simulink model "env_extQ32"  (R2022b)
settings: Solver=VariableStepAuto  StartTime=0.0  StopTime=30  RelTol=1e-3
values from neighbouring files (symbols this model uses):
  B = 8    [variables.m]    (also in variables16.m)
  cordic_delay = 20    [variables.m]    (also in variables16.m)
  e_val = 1/l2    [variables.m]    (also in variables16.m)
  exp_fract_len_homo = 26    [variables.m]    (also in variables16.m = 10)
  exp_word_len_homo = 32    [variables.m]    (also in variables16.m = 16)
  explarge_delay = 3    [variables.m]    (also in variables16.m)
  fft_len_hilb = 2048    [variables.m]    (also in variables16.m)
  fft_length = 4096    [variables.m]    (also in variables16.m)
  frac_bit_l2 = 30    [variables.m]    (also in variables16.m = 14)
  frac_bit_l3 = 29    [variables.m]    (also in variables16.m = 13)
  frac_bit_l4 = 28    [variables.m]    (also in variables16.m = 12)
  grp_delay_hilb = 11    [variables.m]    (also in variables16.m)
  grp_delay_homo = 13    [variables.m]    (also in variables16.m)
  grp_delay_psd = 19    [variables.m]    (also in variables16.m)
  grp_delay_swt = 12    [variables.m]    (also in variables16.m)
  l2 = log(2)    [variables.m]    (also in variables16.m)
  l2e = 1/log2(exp(1))    [variables.m]    (also in variables16.m)
  log2_table = log2((2^(B-1) : 2^(B)) / 2^(B - 1))    [variables.m]    (also in variables16.m)
  log_fract_len_homo = 31    [variables.m]    (also in variables16.m = 15)
  log_latency = 21    [variables.m]    (also in variables16.m)
  log_word_len = 48    [variables.m]    (also in variables16.m = 24)
  log_word_len_homo = 32    [variables.m]    (also in variables16.m = 16)
  NLZLUT = B-ceil(log2((1:2^B)))    [variables.m]    (also in variables16.m)
  scale = 1.0 / (fs * sum(window_val.*window_val))    [variables.m]    (also in variables16.m)
  win_dim = 64    [variables.m]    (also in variables16.m)
  window_dim = 100    [variables.m]    (also in variables16.m)
undefined symbols (not defined in the file or in its folder): c, fl_high_index, fl_low_index, HiD, hilbert_fifo_full, LoD, psd_fifo_full, sfvc784, swt_fifo_full, xck26, xlfda_numerator
libraries: hdlBasic x626, hdlDSPIP x12, hdlUtilities x2, dspsnks4 x1, dspvision x1, vmcUtilities x1
(part 6 of 7)

== system env_extQ32/env_extr/HOMOMORPHIC/log2/normalize_input/stage0 ==
  v_in : Inport
  mem_data_in : Inport  Port=2
  en : Inport  Port=3
  Delay1 : hdlBasic/Delay  rst=off  en=on  latency=1  reg_retiming=off  XmcBlockStatus=1  maskContainerNames=group1  block_type=delay  block_config=sysgen:Delay_config
  Mux : hdlBasic/Mux  inputs=9  en=on  latency=1  precision=Full  arith_type=Unsigned  n_bits=16  bin_pt=14  quantization=Truncate  overflow=Wrap  XmcBlockStatus=1  maskContainerNames=tabcontainer1  block_type=mux  block_config=sysgen:Mux_config
  Reinterpret : hdlBasic/Reinterpret  force_arith_type=on  arith_type=Unsigned  force_bin_pt=on  bin_pt=0  XmcBlockStatus=1  maskContainerNames=group1  block_type=reinterpret  block_config=sysgen:Reinterpret_config
  Shift1 : hdlBasic/Shift  shift_dir=Left  shift_bits=8  en=on  latency=1  precision=Full  arith_type="Signed  (2's comp)"  n_bits=16  bin_pt=14  quantization=Truncate  overflow=Wrap  XmcBlockStatus=1  maskContainerNames=group2  block_type=shift  block_config=sysgen:Shift_config
  Shift2 : hdlBasic/Shift  shift_dir=Left  shift_bits=1  en=on  latency=1  precision=Full  arith_type="Signed  (2's comp)"  n_bits=16  bin_pt=14  quantization=Truncate  overflow=Wrap  XmcBlockStatus=1  maskContainerNames=group2  block_type=shift  block_config=sysgen:Shift_config
  Shift3 : hdlBasic/Shift  shift_dir=Left  shift_bits=2  en=on  latency=1  precision=Full  arith_type="Signed  (2's comp)"  n_bits=16  bin_pt=14  quantization=Truncate  overflow=Wrap  XmcBlockStatus=1  maskContainerNames=group2  block_type=shift  block_config=sysgen:Shift_config
  Shift4 : hdlBasic/Shift  shift_dir=Left  shift_bits=3  en=on  latency=1  precision=Full  arith_type="Signed  (2's comp)"  n_bits=16  bin_pt=14  quantization=Truncate  overflow=Wrap  XmcBlockStatus=1  maskContainerNames=group2  block_type=shift  block_config=sysgen:Shift_config
  Shift5 : hdlBasic/Shift  shift_dir=Left  shift_bits=4  en=on  latency=1  precision=Full  arith_type="Signed  (2's comp)"  n_bits=16  bin_pt=14  quantization=Truncate  overflow=Wrap  XmcBlockStatus=1  maskContainerNames=group2  block_type=shift  block_config=sysgen:Shift_config
  Shift6 : hdlBasic/Shift  shift_dir=Left  shift_bits=5  en=on  latency=1  precision=Full  arith_type="Signed  (2's comp)"  n_bits=16  bin_pt=14  quantization=Truncate  overflow=Wrap  XmcBlockStatus=1  maskContainerNames=group2  block_type=shift  block_config=sysgen:Shift_config
  Shift7 : hdlBasic/Shift  shift_dir=Left  shift_bits=6  en=on  latency=1  precision=Full  arith_type="Signed  (2's comp)"  n_bits=16  bin_pt=14  quantization=Truncate  overflow=Wrap  XmcBlockStatus=1  maskContainerNames=group2  block_type=shift  block_config=sysgen:Shift_config
  Shift8 : hdlBasic/Shift  shift_dir=Left  shift_bits=7  en=on  latency=1  precision=Full  arith_type="Signed  (2's comp)"  n_bits=16  bin_pt=14  quantization=Truncate  overflow=Wrap  XmcBlockStatus=1  maskContainerNames=group2  block_type=shift  block_config=sysgen:Shift_config
  Shift9 : hdlBasic/Shift  shift_dir=Left  shift_bits=0  en=on  latency=1  precision=Full  arith_type="Signed  (2's comp)"  n_bits=16  bin_pt=14  quantization=Truncate  overflow=Wrap  XmcBlockStatus=1  maskContainerNames=group2  block_type=shift  block_config=sysgen:Shift_config
  Slice1 : hdlBasic/Slice  nbits=B  boolean_output=off  mode=Upper Bit Location + Width  bit1=0  base1=MSB of Input  bit0=8  base0=LSB of Input  XmcBlockStatus=1  maskContainerNames=group1  block_type=slice  block_config=sysgen:Slice_config
  v_out : Outport
  n_shift_out : Outport  Port=2
  mem_addr : Outport  Port=3
  wires:
  Shift7/1 -> Mux/8
  v_in/1 -> Reinterpret/1
  Shift4/1 -> Mux/5
  Shift6/1 -> Mux/7
  Shift2/1 -> Mux/3
  Shift8/1 -> Mux/9
  Shift3/1 -> Mux/4
  Shift5/1 -> Mux/6
  Delay1/1 -> n_shift_out/1
  Slice1/1 -> mem_addr/1
  Shift1/1 -> Mux/10
  Reinterpret/1 -> Shift1/1, Shift8/1, Shift7/1, Shift6/1, Shift5/1, Shift4/1, Shift3/1, Shift2/1, Shift9/1, Slice1/1
  Mux/1 -> v_out/1
  mem_data_in/1 -> Delay1/1, Mux/1
  Shift9/1 -> Mux/2
  en/1 -> Shift8/2, Shift7/2, Shift6/2, Shift5/2, Shift3/2, Shift2/2, Delay1/2, Mux/11, Shift9/2, Shift4/2, Shift1/2

== system env_extQ32/env_extr/HOMOMORPHIC/log2/normalize_input/stage1 ==
  v_in : Inport
  n_shift_in : Inport  Port=2
  mem_data_in : Inport  Port=3
  en : Inport  Port=4
  AddSub1 : hdlBasic/AddSub  mode=Addition  use_carryin=off  use_carryout=off  en=on  latency=1  precision=Full  arith_type=Unsigned  n_bits=16  bin_pt=14  quantization=Truncate  overflow=Wrap  use_behavioral_HDL=off  hw_selection=Fabric  pipelined=off  XmcBlockStatus=1  maskContainerNames=tabcontainer1  block_type=addsub  block_config=sysgen:Addsub_config
  Delay2 : hdlBasic/Delay  rst=off  en=on  latency=1  reg_retiming=off  XmcBlockStatus=1  maskContainerNames=group1  block_type=delay  block_config=sysgen:Delay_config
  Mux : hdlBasic/Mux  inputs=9  en=on  latency=1  precision=Full  arith_type=Unsigned  n_bits=16  bin_pt=14  quantization=Truncate  overflow=Wrap  XmcBlockStatus=1  maskContainerNames=tabcontainer1  block_type=mux  block_config=sysgen:Mux_config
  Shift1 : hdlBasic/Shift  shift_dir=Left  shift_bits=8  en=on  latency=1  precision=Full  arith_type="Signed  (2's comp)"  n_bits=16  bin_pt=14  quantization=Truncate  overflow=Wrap  XmcBlockStatus=1  maskContainerNames=group2  block_type=shift  block_config=sysgen:Shift_config
  Shift2 : hdlBasic/Shift  shift_dir=Left  shift_bits=1  en=on  latency=1  precision=Full  arith_type="Signed  (2's comp)"  n_bits=16  bin_pt=14  quantization=Truncate  overflow=Wrap  XmcBlockStatus=1  maskContainerNames=group2  block_type=shift  block_config=sysgen:Shift_config
  Shift3 : hdlBasic/Shift  shift_dir=Left  shift_bits=2  en=on  latency=1  precision=Full  arith_type="Signed  (2's comp)"  n_bits=16  bin_pt=14  quantization=Truncate  overflow=Wrap  XmcBlockStatus=1  maskContainerNames=group2  block_type=shift  block_config=sysgen:Shift_config
  Shift4 : hdlBasic/Shift  shift_dir=Left  shift_bits=3  en=on  latency=1  precision=Full  arith_type="Signed  (2's comp)"  n_bits=16  bin_pt=14  quantization=Truncate  overflow=Wrap  XmcBlockStatus=1  maskContainerNames=group2  block_type=shift  block_config=sysgen:Shift_config
  Shift5 : hdlBasic/Shift  shift_dir=Left  shift_bits=4  en=on  latency=1  precision=Full  arith_type="Signed  (2's comp)"  n_bits=16  bin_pt=14  quantization=Truncate  overflow=Wrap  XmcBlockStatus=1  maskContainerNames=group2  block_type=shift  block_config=sysgen:Shift_config
  Shift6 : hdlBasic/Shift  shift_dir=Left  shift_bits=5  en=on  latency=1  precision=Full  arith_type="Signed  (2's comp)"  n_bits=16  bin_pt=14  quantization=Truncate  overflow=Wrap  XmcBlockStatus=1  maskContainerNames=group2  block_type=shift  block_config=sysgen:Shift_config
  Shift7 : hdlBasic/Shift  shift_dir=Left  shift_bits=6  en=on  latency=1  precision=Full  arith_type="Signed  (2's comp)"  n_bits=16  bin_pt=14  quantization=Truncate  overflow=Wrap  XmcBlockStatus=1  maskContainerNames=group2  block_type=shift  block_config=sysgen:Shift_config
  Shift8 : hdlBasic/Shift  shift_dir=Left  shift_bits=7  en=on  latency=1  precision=Full  arith_type="Signed  (2's comp)"  n_bits=16  bin_pt=14  quantization=Truncate  overflow=Wrap  XmcBlockStatus=1  maskContainerNames=group2  block_type=shift  block_config=sysgen:Shift_config
  Shift9 : hdlBasic/Shift  shift_dir=Left  shift_bits=0  en=on  latency=1  precision=Full  arith_type="Signed  (2's comp)"  n_bits=16  bin_pt=14  quantization=Truncate  overflow=Wrap  XmcBlockStatus=1  maskContainerNames=group2  block_type=shift  block_config=sysgen:Shift_config
  Slice1 : hdlBasic/Slice  nbits=B  boolean_output=off  mode=Upper Bit Location + Width  bit1=0  base1=MSB of Input  bit0=8  base0=LSB of Input  XmcBlockStatus=1  maskContainerNames=group1  block_type=slice  block_config=sysgen:Slice_config
  v_out : Outport
  n_shift_out : Outport  Port=2
  mem_addr : Outport  Port=3
  wires:
  Shift7/1 -> Mux/8
  Shift4/1 -> Mux/5
  Shift6/1 -> Mux/7
  Shift2/1 -> Mux/3
  Shift8/1 -> Mux/9
  Shift3/1 -> Mux/4
  Shift5/1 -> Mux/6
  Slice1/1 -> mem_addr/1
  Shift1/1 -> Mux/10
  v_in/1 -> Shift1/1, Shift8/1, Shift7/1, Shift6/1, Shift5/1, Shift4/1, Shift3/1, Shift2/1, Shift9/1, Slice1/1
  Mux/1 -> v_out/1
  AddSub1/1 -> n_shift_out/1
  n_shift_in/1 -> Delay2/1
  mem_data_in/1 -> AddSub1/2, Mux/1
  Delay2/1 -> AddSub1/1
  Shift9/1 -> Mux/2
  en/1 -> Shift8/2, Shift7/2, Shift6/2, Shift5/2, Shift4/2, Shift3/2, Shift2/2, Mux/11, AddSub1/3, Delay2/2, Shift9/2, Shift1/2

== system env_extQ32/env_extr/HOMOMORPHIC/log2/normalize_input/stage2 ==
  v_in : Inport
  n_shift_in : Inport  Port=2
  mem_data_in : Inport  Port=3
  en : Inport  Port=4
  AddSub1 : hdlBasic/AddSub  mode=Addition  use_carryin=off  use_carryout=off  en=on  latency=1  precision=Full  arith_type=Unsigned  n_bits=16  bin_pt=14  quantization=Truncate  overflow=Wrap  use_behavioral_HDL=off  hw_selection=Fabric  pipelined=off  XmcBlockStatus=1  maskContainerNames=tabcontainer1  block_type=addsub  block_config=sysgen:Addsub_config
  Delay2 : hdlBasic/Delay  rst=off  en=on  latency=1  reg_retiming=off  XmcBlockStatus=1  maskContainerNames=group1  block_type=delay  block_config=sysgen:Delay_config
  Mux : hdlBasic/Mux  inputs=9  en=on  latency=1  precision=Full  arith_type=Unsigned  n_bits=16  bin_pt=14  quantization=Truncate  overflow=Wrap  XmcBlockStatus=1  maskContainerNames=tabcontainer1  block_type=mux  block_config=sysgen:Mux_config
  Shift1 : hdlBasic/Shift  shift_dir=Left  shift_bits=8  en=on  latency=1  precision=Full  arith_type="Signed  (2's comp)"  n_bits=16  bin_pt=14  quantization=Truncate  overflow=Wrap  XmcBlockStatus=1  maskContainerNames=group2  block_type=shift  block_config=sysgen:Shift_config
  Shift2 : hdlBasic/Shift  shift_dir=Left  shift_bits=1  en=on  latency=1  precision=Full  arith_type="Signed  (2's comp)"  n_bits=16  bin_pt=14  quantization=Truncate  overflow=Wrap  XmcBlockStatus=1  maskContainerNames=group2  block_type=shift  block_config=sysgen:Shift_config
  Shift3 : hdlBasic/Shift  shift_dir=Left  shift_bits=2  en=on  latency=1  precision=Full  arith_type="Signed  (2's comp)"  n_bits=16  bin_pt=14  quantization=Truncate  overflow=Wrap  XmcBlockStatus=1  maskContainerNames=group2  block_type=shift  block_config=sysgen:Shift_config
  Shift4 : hdlBasic/Shift  shift_dir=Left  shift_bits=3  en=on  latency=1  precision=Full  arith_type="Signed  (2's comp)"  n_bits=16  bin_pt=14  quantization=Truncate  overflow=Wrap  XmcBlockStatus=1  maskContainerNames=group2  block_type=shift  block_config=sysgen:Shift_config
  Shift5 : hdlBasic/Shift  shift_dir=Left  shift_bits=4  en=on  latency=1  precision=Full  arith_type="Signed  (2's comp)"  n_bits=16  bin_pt=14  quantization=Truncate  overflow=Wrap  XmcBlockStatus=1  maskContainerNames=group2  block_type=shift  block_config=sysgen:Shift_config
  Shift6 : hdlBasic/Shift  shift_dir=Left  shift_bits=5  en=on  latency=1  precision=Full  arith_type="Signed  (2's comp)"  n_bits=16  bin_pt=14  quantization=Truncate  overflow=Wrap  XmcBlockStatus=1  maskContainerNames=group2  block_type=shift  block_config=sysgen:Shift_config
  Shift7 : hdlBasic/Shift  shift_dir=Left  shift_bits=6  en=on  latency=1  precision=Full  arith_type="Signed  (2's comp)"  n_bits=16  bin_pt=14  quantization=Truncate  overflow=Wrap  XmcBlockStatus=1  maskContainerNames=group2  block_type=shift  block_config=sysgen:Shift_config
  Shift8 : hdlBasic/Shift  shift_dir=Left  shift_bits=7  en=on  latency=1  precision=Full  arith_type="Signed  (2's comp)"  n_bits=16  bin_pt=14  quantization=Truncate  overflow=Wrap  XmcBlockStatus=1  maskContainerNames=group2  block_type=shift  block_config=sysgen:Shift_config
  Shift9 : hdlBasic/Shift  shift_dir=Left  shift_bits=0  en=on  latency=1  precision=Full  arith_type="Signed  (2's comp)"  n_bits=16  bin_pt=14  quantization=Truncate  overflow=Wrap  XmcBlockStatus=1  maskContainerNames=group2  block_type=shift  block_config=sysgen:Shift_config
  Slice1 : hdlBasic/Slice  nbits=B  boolean_output=off  mode=Upper Bit Location + Width  bit1=0  base1=MSB of Input  bit0=8  base0=LSB of Input  XmcBlockStatus=1  maskContainerNames=group1  block_type=slice  block_config=sysgen:Slice_config
  v_out : Outport
  n_shift_out : Outport  Port=2
  mem_addr : Outport  Port=3
  wires:
  Shift7/1 -> Mux/8
  Shift4/1 -> Mux/5
  Shift6/1 -> Mux/7
  Shift2/1 -> Mux/3
  Shift8/1 -> Mux/9
  Shift3/1 -> Mux/4
  Shift5/1 -> Mux/6
  Slice1/1 -> mem_addr/1
  Shift1/1 -> Mux/10
  v_in/1 -> Shift1/1, Shift8/1, Shift7/1, Shift6/1, Shift5/1, Shift4/1, Shift3/1, Shift2/1, Shift9/1, Slice1/1
  Mux/1 -> v_out/1
  AddSub1/1 -> n_shift_out/1
  n_shift_in/1 -> Delay2/1
  mem_data_in/1 -> AddSub1/2, Mux/1
  Delay2/1 -> AddSub1/1
  Shift9/1 -> Mux/2
  en/1 -> Shift8/2, Shift7/2, Shift6/2, Shift5/2, Shift4/2, Shift3/2, Shift2/2, Delay2/2, Mux/11, AddSub1/3, Shift9/2, Shift1/2

== system env_extQ32/env_extr/HOMOMORPHIC/log2/normalize_input/stage3 ==
  v_in : Inport
  n_shift_in : Inport  Port=2
  mem_data_in : Inport  Port=3
  en : Inport  Port=4
  AddSub1 : hdlBasic/AddSub  mode=Subtraction  use_carryin=off  use_carryout=off  en=on  latency=1  precision=Full  arith_type=Unsigned  n_bits=16  bin_pt=14  quantization=Truncate  overflow=Wrap  use_behavioral_HDL=off  hw_selection=Fabric  pipelined=off  XmcBlockStatus=1  maskContainerNames=tabcontainer1  block_type=addsub  block_config=sysgen:Addsub_config
  AddSub2 : hdlBasic/AddSub  mode=Subtraction  use_carryin=off  use_carryout=off  en=on  latency=1  precision=Full  arith_type=Unsigned  n_bits=16  bin_pt=14  quantization=Truncate  overflow=Wrap  use_behavioral_HDL=off  hw_selection=Fabric  pipelined=off  XmcBlockStatus=1  maskContainerNames=tabcontainer1  block_type=addsub  block_config=sysgen:Addsub_config
  Constant1 : hdlBasic/Constant  const=log_word_len_homo-log_fract_len_homo-1  gui_display_data_type=Fixed-point  arith_type=Unsigned  n_bits=ceil(log2(log_word_len_homo-log_fract_len_homo+1))  bin_pt=0  preci_type=Single  exp_width=8  frac_width=24  explicit_period=off  period=1  XmcBlockStatus=1  maskContainerNames=tabcontainer1  block_type=constant  block_config=sysgen:Constant_config
  Mux : hdlBasic/Mux  inputs=9  en=on  latency=1  precision=Full  arith_type=Unsigned  n_bits=16  bin_pt=14  quantization=Truncate  overflow=Wrap  XmcBlockStatus=1  maskContainerNames=tabcontainer1  block_type=mux  block_config=sysgen:Mux_config
  Reinterpret : hdlBasic/Reinterpret  force_arith_type=off  arith_type=Unsigned  force_bin_pt=on  bin_pt=log_word_len_homo-1  XmcBlockStatus=1  maskContainerNames=group1  block_type=reinterpret  block_config=sysgen:Reinterpret_config
  Shift1 : hdlBasic/Shift  shift_dir=Left  shift_bits=8  en=on  latency=1  precision=Full  arith_type="Signed  (2's comp)"  n_bits=16  bin_pt=14  quantization=Truncate  overflow=Wrap  XmcBlockStatus=1  maskContainerNames=group2  block_type=shift  block_config=sysgen:Shift_config
  Shift2 : hdlBasic/Shift  shift_dir=Left  shift_bits=1  en=on  latency=1  precision=Full  arith_type="Signed  (2's comp)"  n_bits=16  bin_pt=14  quantization=Truncate  overflow=Wrap  XmcBlockStatus=1  maskContainerNames=group2  block_type=shift  block_config=sysgen:Shift_config
  Shift3 : hdlBasic/Shift  shift_dir=Left  shift_bits=2  en=on  latency=1  precision=Full  arith_type="Signed  (2's comp)"  n_bits=16  bin_pt=14  quantization=Truncate  overflow=Wrap  XmcBlockStatus=1  maskContainerNames=group2  block_type=shift  block_config=sysgen:Shift_config
  Shift4 : hdlBasic/Shift  shift_dir=Left  shift_bits=3  en=on  latency=1  precision=Full  arith_type="Signed  (2's comp)"  n_bits=16  bin_pt=14  quantization=Truncate  overflow=Wrap  XmcBlockStatus=1  maskContainerNames=group2  block_type=shift  block_config=sysgen:Shift_config
  Shift5 : hdlBasic/Shift  shift_dir=Left  shift_bits=4  en=on  latency=1  precision=Full  arith_type="Signed  (2's comp)"  n_bits=16  bin_pt=14  quantization=Truncate  overflow=Wrap  XmcBlockStatus=1  maskContainerNames=group2  block_type=shift  block_config=sysgen:Shift_config
  Shift6 : hdlBasic/Shift  shift_dir=Left  shift_bits=5  en=on  latency=1  precision=Full  arith_type="Signed  (2's comp)"  n_bits=16  bin_pt=14  quantization=Truncate  overflow=Wrap  XmcBlockStatus=1  maskContainerNames=group2  block_type=shift  block_config=sysgen:Shift_config
  Shift7 : hdlBasic/Shift  shift_dir=Left  shift_bits=6  en=on  latency=1  precision=Full  arith_type="Signed  (2's comp)"  n_bits=16  bin_pt=14  quantization=Truncate  overflow=Wrap  XmcBlockStatus=1  maskContainerNames=group2  block_type=shift  block_config=sysgen:Shift_config
  Shift8 : hdlBasic/Shift  shift_dir=Left  shift_bits=7  en=on  latency=1  precision=Full  arith_type="Signed  (2's comp)"  n_bits=16  bin_pt=14  quantization=Truncate  overflow=Wrap  XmcBlockStatus=1  maskContainerNames=group2  block_type=shift  block_config=sysgen:Shift_config
  Shift9 : hdlBasic/Shift  shift_dir=Left  shift_bits=0  en=on  latency=1  precision=Full  arith_type="Signed  (2's comp)"  n_bits=16  bin_pt=14  quantization=Truncate  overflow=Wrap  XmcBlockStatus=1  maskContainerNames=group2  block_type=shift  block_config=sysgen:Shift_config
  Slice1 : hdlBasic/Slice  nbits=B  boolean_output=off  mode=Upper Bit Location + Width  bit1=0  base1=MSB of Input  bit0=8  base0=LSB of Input  XmcBlockStatus=1  maskContainerNames=group1  block_type=slice  block_config=sysgen:Slice_config
  v_out : Outport
  n_shift_out : Outport  Port=2
  mem_addr : Outport  Port=3
  wires:
  Shift7/1 -> Mux/8
  Shift4/1 -> Mux/5
  Shift6/1 -> Mux/7
  Shift2/1 -> Mux/3
  Shift8/1 -> Mux/9
  Shift3/1 -> Mux/4
  Shift5/1 -> Mux/6
  Mux/1 -> Reinterpret/1
  n_shift_in/1 -> AddSub2/2
  AddSub2/1 -> AddSub1/1
  Constant1/1 -> AddSub2/1
  mem_data_in/1 -> AddSub1/2, Mux/1
  v_in/1 -> Slice1/1, Shift1/1, Shift8/1, Shift7/1, Shift6/1, Shift5/1, Shift4/1, Shift3/1, Shift2/1, Shift9/1
  Slice1/1 -> mem_addr/1
  Reinterpret/1 -> v_out/1
  Shift1/1 -> Mux/10
  AddSub1/1 -> n_shift_out/1
  Shift9/1 -> Mux/2
  en/1 -> Shift8/2, Shift7/2, Shift6/2, Shift5/2, Shift4/2, Shift3/2, Shift2/2, AddSub2/3, Mux/11, AddSub1/3, Shift9/2, Shift1/2

== system env_extQ32/env_extr/SWT/shannonE/log2/normalize_input ==
  data_in : Inport
  en : Inport  Port=2
  Constant1 : hdlBasic/Constant  const=0  gui_display_data_type=Boolean  arith_type=Boolean  n_bits=16  bin_pt=14  preci_type=Single  exp_width=8  frac_width=24  explicit_period=off  period=1  XmcBlockStatus=1  maskContainerNames=tabcontainer1  block_type=constant  block_config=sysgen:Constant_config
  Constant2 : hdlBasic/Constant  const=0  gui_display_data_type=Boolean  arith_type=Boolean  n_bits=16  bin_pt=14  preci_type=Single  exp_width=8  frac_width=24  explicit_period=off  period=1  XmcBlockStatus=1  maskContainerNames=tabcontainer1  block_type=constant  block_config=sysgen:Constant_config
  Constant3 : hdlBasic/Constant  const=0  gui_display_data_type=Fixed-point  arith_type=Unsigned  n_bits=ceil(log2(B)+1)  bin_pt=0  preci_type=Single  exp_width=8  frac_width=24  explicit_period=off  period=1  XmcBlockStatus=1  maskContainerNames=tabcontainer1  block_type=constant  block_config=sysgen:Constant_config
  Constant4 : hdlBasic/Constant  const=0  gui_display_data_type=Fixed-point  arith_type=Unsigned  n_bits=ceil(log2(B)+1)  bin_pt=0  preci_type=Single  exp_width=8  frac_width=24  explicit_period=off  period=1  XmcBlockStatus=1  maskContainerNames=tabcontainer1  block_type=constant  block_config=sysgen:Constant_config
  Constant7 : hdlBasic/Constant  const=0  gui_display_data_type=Boolean  arith_type=Boolean  n_bits=16  bin_pt=14  preci_type=Single  exp_width=8  frac_width=24  explicit_period=off  period=1  XmcBlockStatus=1  maskContainerNames=tabcontainer1  block_type=constant  block_config=sysgen:Constant_config
  Constant8 : hdlBasic/Constant  const=0  gui_display_data_type=Fixed-point  arith_type=Unsigned  n_bits=ceil(log2(B)+1)  bin_pt=0  preci_type=Single  exp_width=8  frac_width=24  explicit_period=off  period=1  XmcBlockStatus=1  maskContainerNames=tabcontainer1  block_type=constant  block_config=sysgen:Constant_config
  Dual Port RAM : hdlBasic/Dual Port RAM  depth=length(NLZLUT)  initVector=NLZLUT  distributed_mem=Block RAM  init_a=0  init_b=0  rst_a=off  rst_b=off  en_a=on  en_b=on  latency=1  write_mode_A=Read After Write  write_mode_B=Read After Write  explicit_period=[]  period=[]  simulation_type=fast_sim  XmcBlockStatus=1  maskContainerNames=tabcontainer1  block_type=dpram  block_config=sysgen:Dpram_config  optimize=Area
      settings: infoedit=[]
  Dual Port RAM1 : hdlBasic/Dual Port RAM  depth=length(NLZLUT)  initVector=NLZLUT  distributed_mem=Block RAM  init_a=0  init_b=0  rst_a=off  rst_b=off  en_a=on  en_b=on  latency=1  write_mode_A=Read After Write  write_mode_B=Read After Write  explicit_period=[]  period=[]  simulation_type=fast_sim  XmcBlockStatus=1  maskContainerNames=tabcontainer1  block_type=dpram  block_config=sysgen:Dpram_config  optimize=Area
      settings: infoedit=[]
  Dual Port RAM3 : hdlBasic/Dual Port RAM  depth=length(NLZLUT)  initVector=NLZLUT  distributed_mem=Block RAM  init_a=0  init_b=0  rst_a=off  rst_b=off  en_a=on  en_b=on  latency=1  write_mode_A=Read After Write  write_mode_B=Read After Write  explicit_period=[]  period=[]  simulation_type=fast_sim  XmcBlockStatus=1  maskContainerNames=tabcontainer1  block_type=dpram  block_config=sysgen:Dpram_config  optimize=Area
      settings: infoedit=[]
  stage0 : Subsystem
      settings: PortSchema="{\"entries\":[{\"content\":{\"sides\":[{\"content\":{\"connectorIds\":[\"In1\"]},\"type\":\"ConnectorPlacement.EquallySpacedRectSide\",\"uuid\":\"2efcf317-0d6c-449c-9b5f-ecffd8c2580d\"},{\"content\":{\"connectorIds\":[\"Out1\",\"Out2\"],\"side\":\"RIGHT\"},\"type\":\"ConnectorPlacement.EquallySpacedRectSide\",\"uuid\":\"64d64660-0707-42f2-9c9c-1ef5504f52ac\"},{\"content\":{\"connectorIds\":[\"In2\",\"In3\",\"Out3\"],\"side\":\"TOP\"},\"type\":\"ConnectorPlacement.EquallySpacedRectSide\",\"uuid\":\"46f06ac4-fdd0-4e37-81b8-c7ff4ab208c3\"}]},\"type\":\"ConnectorPlacement.EquallySpacedConnector\",\"uuid\":\"22d944fc-118c-4e93-8f45-ec21c3a091f8\"}],\"packageUris\":[\"http://schema.mathworks.com/mf0/Connector/R2020b\"],\"version\":\"1.0\"}"
  stage1 : Subsystem
      settings: PortSchema="{\"entries\":[{\"content\":{\"sides\":[{\"content\":{\"connectorIds\":[\"In1\",\"In2\"]},\"type\":\"ConnectorPlacement.EquallySpacedRectSide\",\"uuid\":\"9d039a16-3a48-49d5-80b7-ade04a8e7f96\"},{\"content\":{\"connectorIds\":[\"Out1\",\"Out2\"],\"side\":\"RIGHT\"},\"type\":\"ConnectorPlacement.EquallySpacedRectSide\",\"uuid\":\"bb4be220-296c-4d2d-b90e-a958a467eb47\"},{\"content\":{\"connectorIds\":[\"In3\",\"In4\",\"Out3\"],\"side\":\"TOP\"},\"type\":\"ConnectorPlacement.EquallySpacedRectSide\",\"uuid\":\"bb4a24ca-25c4-4b34-8f6b-74df8c85655a\"}]},\"type\":\"ConnectorPlacement.EquallySpacedConnector\",\"uuid\":\"a2ca7259-7cd6-4f5b-b082-7ba40fce56a8\"}],\"packageUris\":[\"http://schema.mathworks.com/mf0/Connector/R2020b\"],\"version\":\"1.0\"}"
  stage2 : Subsystem
      settings: PortSchema="{\"entries\":[{\"content\":{\"sides\":[{\"content\":{\"connectorIds\":[\"In1\",\"In2\"]},\"type\":\"ConnectorPlacement.EquallySpacedRectSide\",\"uuid\":\"9d039a16-3a48-49d5-80b7-ade04a8e7f96\"},{\"content\":{\"connectorIds\":[\"Out1\",\"Out2\"],\"side\":\"RIGHT\"},\"type\":\"ConnectorPlacement.EquallySpacedRectSide\",\"uuid\":\"bb4be220-296c-4d2d-b90e-a958a467eb47\"},{\"content\":{\"connectorIds\":[\"In3\",\"In4\",\"Out3\"],\"side\":\"TOP\"},\"type\":\"ConnectorPlacement.EquallySpacedRectSide\",\"uuid\":\"bb4a24ca-25c4-4b34-8f6b-74df8c85655a\"}]},\"type\":\"ConnectorPlacement.EquallySpacedConnector\",\"uuid\":\"a2ca7259-7cd6-4f5b-b082-7ba40fce56a8\"}],\"packageUris\":[\"http://schema.mathworks.com/mf0/Connector/R2020b\"],\"version\":\"1.0\"}"
  stage3 : Subsystem
      settings: PortSchema="{\"entries\":[{\"content\":{\"sides\":[{\"content\":{\"connectorIds\":[\"In1\",\"In2\"]},\"type\":\"ConnectorPlacement.EquallySpacedRectSide\",\"uuid\":\"9d039a16-3a48-49d5-80b7-ade04a8e7f96\"},{\"content\":{\"connectorIds\":[\"Out1\",\"Out2\"],\"side\":\"RIGHT\"},\"type\":\"ConnectorPlacement.EquallySpacedRectSide\",\"uuid\":\"bb4be220-296c-4d2d-b90e-a958a467eb47\"},{\"content\":{\"connectorIds\":[\"In3\",\"In4\",\"Out3\"],\"side\":\"TOP\"},\"type\":\"ConnectorPlacement.EquallySpacedRectSide\",\"uuid\":\"bb4a24ca-25c4-4b34-8f6b-74df8c85655a\"}]},\"type\":\"ConnectorPlacement.EquallySpacedConnector\",\"uuid\":\"a2ca7259-7cd6-4f5b-b082-7ba40fce56a8\"}],\"packageUris\":[\"http://schema.mathworks.com/mf0/Connector/R2020b\"],\"version\":\"1.0\"}"
  stage7 : Subsystem
      settings: PortSchema="{\"entries\":[{\"content\":{\"sides\":[{\"content\":{\"connectorIds\":[\"In1\",\"In2\"]},\"type\":\"ConnectorPlacement.EquallySpacedRectSide\",\"uuid\":\"9d039a16-3a48-49d5-80b7-ade04a8e7f96\"},{\"content\":{\"connectorIds\":[\"Out1\",\"Out2\"],\"side\":\"RIGHT\"},\"type\":\"ConnectorPlacement.EquallySpacedRectSide\",\"uuid\":\"bb4be220-296c-4d2d-b90e-a958a467eb47\"},{\"content\":{\"connectorIds\":[\"In3\",\"In4\",\"Out3\"],\"side\":\"TOP\"},\"type\":\"ConnectorPlacement.EquallySpacedRectSide\",\"uuid\":\"bb4a24ca-25c4-4b34-8f6b-74df8c85655a\"}]},\"type\":\"ConnectorPlacement.EquallySpacedConnector\",\"uuid\":\"a2ca7259-7cd6-4f5b-b082-7ba40fce56a8\"}],\"packageUris\":[\"http://schema.mathworks.com/mf0/Connector/R2020b\"],\"version\":\"1.0\"}"
  stage8 : Subsystem
      settings: PortSchema="{\"entries\":[{\"content\":{\"sides\":[{\"content\":{\"connectorIds\":[\"In1\",\"In2\"]},\"type\":\"ConnectorPlacement.EquallySpacedRectSide\",\"uuid\":\"f634d078-23dc-4ab7-95a0-12deec3a8dc3\"},{\"content\":{\"connectorIds\":[\"Out1\",\"Out2\"],\"side\":\"RIGHT\"},\"type\":\"ConnectorPlacement.EquallySpacedRectSide\",\"uuid\":\"3b518452-2987-4406-a2e9-8ddbf9d6e9f5\"},{\"content\":{\"connectorIds\":[\"In3\",\"In4\",\"Out3\"],\"side\":\"TOP\"},\"type\":\"ConnectorPlacement.EquallySpacedRectSide\",\"uuid\":\"9ad2e8b0-6de8-48f9-a4db-ba88e5ff6307\"}]},\"type\":\"ConnectorPlacement.EquallySpacedConnector\",\"uuid\":\"bfdc1522-4211-4337-893d-197f1173dc35\"}],\"packageUris\":[\"http://schema.mathworks.com/mf0/Connector/R2020b\"],\"version\":\"1.0\"}"
  data_out_x : Outport
  data_out_n : Outport  Port=2
  wires:
  stage8/1(v_out) -> data_out_x/1
  stage8/2(n_shift_out) -> data_out_n/1
  stage7/1(v_out) -> stage8/1(v_in)
  stage7/2(n_shift_out) -> stage8/2(n_shift_in)
  data_in/1 -> stage0/1(v_in)
  stage0/1(v_out) -> stage1/1(v_in)
  stage0/2(n_shift_out) -> stage1/2(n_shift_in)
  Constant2/1 -> Dual Port RAM/3, Dual Port RAM/6
  Constant3/1 -> Dual Port RAM/2, Dual Port RAM/5
  Dual Port RAM/1 -> stage0/2(mem_data_in)  "log2lut"
  stage0/3(mem_addr) -> Dual Port RAM/1
  Dual Port RAM/2 -> stage1/3(mem_data_in)  "log2luti1"
  stage1/3(mem_addr) -> Dual Port RAM/4
  Constant7/1 -> Dual Port RAM3/3, Dual Port RAM3/6
  Constant8/1 -> Dual Port RAM3/5, Dual Port RAM3/2
  Dual Port RAM3/2 -> stage7/3(mem_data_in)  "log2luti1"
  stage7/3(mem_addr) -> Dual Port RAM3/4
  Dual Port RAM3/1 -> stage8/3(mem_data_in)  "log2lut"
  stage8/3(mem_addr) -> Dual Port RAM3/1
  stage2/1(v_out) -> stage3/1(v_in)
  stage2/2(n_shift_out) -> stage3/2(n_shift_in)
  stage1/1(v_out) -> stage2/1(v_in)
  stage1/2(n_shift_out) -> stage2/2(n_shift_in)
  stage3/2(n_shift_out) -> stage7/2(n_shift_in)
  stage3/1(v_out) -> stage7/1(v_in)
  en/1 -> Dual Port RAM1/8, Dual Port RAM1/7, stage3/4(en), stage7/4(en), Dual Port RAM3/8, Dual Port RAM3/7, stage8/4(en), stage2/4(en), stage1/4(en), Dual Port RAM/8, Dual Port RAM/7, stage0/3(en)
  Constant4/1 -> Dual Port RAM1/2, Dual Port RAM1/5
  Constant1/1 -> Dual Port RAM1/3, Dual Port RAM1/6
  stage2/3(mem_addr) -> Dual Port RAM1/1
  Dual Port RAM1/1 -> stage2/3(mem_data_in)  "log2lut"
  Dual Port RAM1/2 -> stage3/3(mem_data_in)  "log2luti1"
  stage3/3(mem_addr) -> Dual Port RAM1/4

== system env_extQ32/env_extr/SWT/shannonE/log2/normalize_input/stage0 ==
  v_in : Inport
  mem_data_in : Inport  Port=2
  en : Inport  Port=3
  Delay1 : hdlBasic/Delay  rst=off  en=on  latency=1  reg_retiming=off  XmcBlockStatus=1  maskContainerNames=group1  block_type=delay  block_config=sysgen:Delay_config
  Mux : hdlBasic/Mux  inputs=9  en=on  latency=1  precision=Full  arith_type=Unsigned  n_bits=16  bin_pt=14  quantization=Truncate  overflow=Wrap  XmcBlockStatus=1  maskContainerNames=tabcontainer1  block_type=mux  block_config=sysgen:Mux_config
  ROM : hdlBasic/ROM  Commented=on  depth=length(NLZLUT)  initVector=NLZLUT  distributed_mem=Block RAM  rst=off  init_reg=0  en=off  latency=1  gui_display_data_type=Fixed-point  arith_type=Unsigned  n_bits=ceil(log2(B)+1)  bin_pt=0  preci_type=Single  exp_width=8  frac_width=24  optimize=Area  use_rpm=on  simulation_type=fast_sim  XmcBlockStatus=1  maskContainerNames=tabcontainer1  block_type=sprom  block_config=sysgen:SPROM_config
  Reinterpret : hdlBasic/Reinterpret  force_arith_type=on  arith_type=Unsigned  force_bin_pt=on  bin_pt=0  XmcBlockStatus=1  maskContainerNames=group1  block_type=reinterpret  block_config=sysgen:Reinterpret_config
  Shift1 : hdlBasic/Shift  shift_dir=Left  shift_bits=8  en=on  latency=1  precision=Full  arith_type="Signed  (2's comp)"  n_bits=16  bin_pt=14  quantization=Truncate  overflow=Wrap  XmcBlockStatus=1  maskContainerNames=group2  block_type=shift  block_config=sysgen:Shift_config
  Shift2 : hdlBasic/Shift  shift_dir=Left  shift_bits=1  en=on  latency=1  precision=Full  arith_type="Signed  (2's comp)"  n_bits=16  bin_pt=14  quantization=Truncate  overflow=Wrap  XmcBlockStatus=1  maskContainerNames=group2  block_type=shift  block_config=sysgen:Shift_config
  Shift3 : hdlBasic/Shift  shift_dir=Left  shift_bits=2  en=on  latency=1  precision=Full  arith_type="Signed  (2's comp)"  n_bits=16  bin_pt=14  quantization=Truncate  overflow=Wrap  XmcBlockStatus=1  maskContainerNames=group2  block_type=shift  block_config=sysgen:Shift_config
  Shift4 : hdlBasic/Shift  shift_dir=Left  shift_bits=3  en=on  latency=1  precision=Full  arith_type="Signed  (2's comp)"  n_bits=16  bin_pt=14  quantization=Truncate  overflow=Wrap  XmcBlockStatus=1  maskContainerNames=group2  block_type=shift  block_config=sysgen:Shift_config
  Shift5 : hdlBasic/Shift  shift_dir=Left  shift_bits=4  en=on  latency=1  precision=Full  arith_type="Signed  (2's comp)"  n_bits=16  bin_pt=14  quantization=Truncate  overflow=Wrap  XmcBlockStatus=1  maskContainerNames=group2  block_type=shift  block_config=sysgen:Shift_config
  Shift6 : hdlBasic/Shift  shift_dir=Left  shift_bits=5  en=on  latency=1  precision=Full  arith_type="Signed  (2's comp)"  n_bits=16  bin_pt=14  quantization=Truncate  overflow=Wrap  XmcBlockStatus=1  maskContainerNames=group2  block_type=shift  block_config=sysgen:Shift_config
  Shift7 : hdlBasic/Shift  shift_dir=Left  shift_bits=6  en=on  latency=1  precision=Full  arith_type="Signed  (2's comp)"  n_bits=16  bin_pt=14  quantization=Truncate  overflow=Wrap  XmcBlockStatus=1  maskContainerNames=group2  block_type=shift  block_config=sysgen:Shift_config
  Shift8 : hdlBasic/Shift  shift_dir=Left  shift_bits=7  en=on  latency=1  precision=Full  arith_type="Signed  (2's comp)"  n_bits=16  bin_pt=14  quantization=Truncate  overflow=Wrap  XmcBlockStatus=1  maskContainerNames=group2  block_type=shift  block_config=sysgen:Shift_config
  Shift9 : hdlBasic/Shift  shift_dir=Left  shift_bits=0  en=on  latency=1  precision=Full  arith_type="Signed  (2's comp)"  n_bits=16  bin_pt=14  quantization=Truncate  overflow=Wrap  XmcBlockStatus=1  maskContainerNames=group2  block_type=shift  block_config=sysgen:Shift_config
  Slice1 : hdlBasic/Slice  nbits=B  boolean_output=off  mode=Upper Bit Location + Width  bit1=0  base1=MSB of Input  bit0=8  base0=LSB of Input  XmcBlockStatus=1  maskContainerNames=group1  block_type=slice  block_config=sysgen:Slice_config
  v_out : Outport
  n_shift_out : Outport  Port=2
  mem_addr : Outport  Port=3
  wires:
  Shift7/1 -> Mux/8
  v_in/1 -> Reinterpret/1
  Shift4/1 -> Mux/5
  Shift6/1 -> Mux/7
  Shift2/1 -> Mux/3
  Shift8/1 -> Mux/9
  Shift3/1 -> Mux/4
  Shift5/1 -> Mux/6
  Delay1/1 -> n_shift_out/1
  Slice1/1 -> mem_addr/1
  Shift1/1 -> Mux/10
  Reinterpret/1 -> Shift1/1, Shift8/1, Shift7/1, Shift6/1, Shift5/1, Shift4/1, Shift3/1, Shift2/1, Shift9/1, Slice1/1
  Mux/1 -> v_out/1
  mem_data_in/1 -> Delay1/1, Mux/1
  Shift9/1 -> Mux/2
  en/1 -> Mux/11, Delay1/2, Shift9/2, Shift2/2, Shift3/2, Shift4/2, Shift5/2, Shift6/2, Shift7/2, Shift8/2, Shift1/2

== system env_extQ32/env_extr/SWT/shannonE/log2/normalize_input/stage1 ==
  v_in : Inport
  n_shift_in : Inport  Port=2
  mem_data_in : Inport  Port=3
  en : Inport  Port=4
  AddSub1 : hdlBasic/AddSub  mode=Addition  use_carryin=off  use_carryout=off  en=on  latency=1  precision=Full  arith_type=Unsigned  n_bits=16  bin_pt=14  quantization=Truncate  overflow=Wrap  use_behavioral_HDL=off  hw_selection=Fabric  pipelined=off  XmcBlockStatus=1  maskContainerNames=tabcontainer1  block_type=addsub  block_config=sysgen:Addsub_config
  Delay2 : hdlBasic/Delay  rst=off  en=on  latency=1  reg_retiming=off  XmcBlockStatus=1  maskContainerNames=group1  block_type=delay  block_config=sysgen:Delay_config
  Mux : hdlBasic/Mux  inputs=9  en=on  latency=1  precision=Full  arith_type=Unsigned  n_bits=16  bin_pt=14  quantization=Truncate  overflow=Wrap  XmcBlockStatus=1  maskContainerNames=tabcontainer1  block_type=mux  block_config=sysgen:Mux_config
  Shift1 : hdlBasic/Shift  shift_dir=Left  shift_bits=8  en=on  latency=1  precision=Full  arith_type="Signed  (2's comp)"  n_bits=16  bin_pt=14  quantization=Truncate  overflow=Wrap  XmcBlockStatus=1  maskContainerNames=group2  block_type=shift  block_config=sysgen:Shift_config
  Shift2 : hdlBasic/Shift  shift_dir=Left  shift_bits=1  en=on  latency=1  precision=Full  arith_type="Signed  (2's comp)"  n_bits=16  bin_pt=14  quantization=Truncate  overflow=Wrap  XmcBlockStatus=1  maskContainerNames=group2  block_type=shift  block_config=sysgen:Shift_config
  Shift3 : hdlBasic/Shift  shift_dir=Left  shift_bits=2  en=on  latency=1  precision=Full  arith_type="Signed  (2's comp)"  n_bits=16  bin_pt=14  quantization=Truncate  overflow=Wrap  XmcBlockStatus=1  maskContainerNames=group2  block_type=shift  block_config=sysgen:Shift_config
  Shift4 : hdlBasic/Shift  shift_dir=Left  shift_bits=3  en=on  latency=1  precision=Full  arith_type="Signed  (2's comp)"  n_bits=16  bin_pt=14  quantization=Truncate  overflow=Wrap  XmcBlockStatus=1  maskContainerNames=group2  block_type=shift  block_config=sysgen:Shift_config
  Shift5 : hdlBasic/Shift  shift_dir=Left  shift_bits=4  en=on  latency=1  precision=Full  arith_type="Signed  (2's comp)"  n_bits=16  bin_pt=14  quantization=Truncate  overflow=Wrap  XmcBlockStatus=1  maskContainerNames=group2  block_type=shift  block_config=sysgen:Shift_config
  Shift6 : hdlBasic/Shift  shift_dir=Left  shift_bits=5  en=on  latency=1  precision=Full  arith_type="Signed  (2's comp)"  n_bits=16  bin_pt=14  quantization=Truncate  overflow=Wrap  XmcBlockStatus=1  maskContainerNames=group2  block_type=shift  block_config=sysgen:Shift_config
  Shift7 : hdlBasic/Shift  shift_dir=Left  shift_bits=6  en=on  latency=1  precision=Full  arith_type="Signed  (2's comp)"  n_bits=16  bin_pt=14  quantization=Truncate  overflow=Wrap  XmcBlockStatus=1  maskContainerNames=group2  block_type=shift  block_config=sysgen:Shift_config
  Shift8 : hdlBasic/Shift  shift_dir=Left  shift_bits=7  en=on  latency=1  precision=Full  arith_type="Signed  (2's comp)"  n_bits=16  bin_pt=14  quantization=Truncate  overflow=Wrap  XmcBlockStatus=1  maskContainerNames=group2  block_type=shift  block_config=sysgen:Shift_config
  Shift9 : hdlBasic/Shift  shift_dir=Left  shift_bits=0  en=on  latency=1  precision=Full  arith_type="Signed  (2's comp)"  n_bits=16  bin_pt=14  quantization=Truncate  overflow=Wrap  XmcBlockStatus=1  maskContainerNames=group2  block_type=shift  block_config=sysgen:Shift_config
  Slice1 : hdlBasic/Slice  nbits=B  boolean_output=off  mode=Upper Bit Location + Width  bit1=0  base1=MSB of Input  bit0=8  base0=LSB of Input  XmcBlockStatus=1  maskContainerNames=group1  block_type=slice  block_config=sysgen:Slice_config
  v_out : Outport
  n_shift_out : Outport  Port=2
  mem_addr : Outport  Port=3
  wires:
  Shift7/1 -> Mux/8
  Shift4/1 -> Mux/5
  Shift6/1 -> Mux/7
  Shift2/1 -> Mux/3
  Shift8/1 -> Mux/9
  Shift3/1 -> Mux/4
  Shift5/1 -> Mux/6
  Slice1/1 -> mem_addr/1
  Shift1/1 -> Mux/10
  v_in/1 -> Shift1/1, Shift8/1, Shift7/1, Shift6/1, Shift5/1, Shift4/1, Shift3/1, Shift2/1, Shift9/1, Slice1/1
  Mux/1 -> v_out/1
  AddSub1/1 -> n_shift_out/1
  n_shift_in/1 -> Delay2/1
  mem_data_in/1 -> AddSub1/2, Mux/1
  Delay2/1 -> AddSub1/1
  Shift9/1 -> Mux/2
  en/1 -> Shift7/2, Shift6/2, Shift5/2, Shift4/2, Shift3/2, Shift2/2, Mux/11, AddSub1/3, Delay2/2, Shift9/2, Shift8/2, Shift1/2

== system env_extQ32/env_extr/SWT/shannonE/log2/normalize_input/stage2 ==
  v_in : Inport
  n_shift_in : Inport  Port=2
  mem_data_in : Inport  Port=3
  en : Inport  Port=4
  AddSub1 : hdlBasic/AddSub  mode=Addition  use_carryin=off  use_carryout=off  en=on  latency=1  precision=Full  arith_type=Unsigned  n_bits=16  bin_pt=14  quantization=Truncate  overflow=Wrap  use_behavioral_HDL=off  hw_selection=Fabric  pipelined=off  XmcBlockStatus=1  maskContainerNames=tabcontainer1  block_type=addsub  block_config=sysgen:Addsub_config
  Delay2 : hdlBasic/Delay  rst=off  en=on  latency=1  reg_retiming=off  XmcBlockStatus=1  maskContainerNames=group1  block_type=delay  block_config=sysgen:Delay_config
  Mux : hdlBasic/Mux  inputs=9  en=on  latency=1  precision=Full  arith_type=Unsigned  n_bits=16  bin_pt=14  quantization=Truncate  overflow=Wrap  XmcBlockStatus=1  maskContainerNames=tabcontainer1  block_type=mux  block_config=sysgen:Mux_config
  Shift1 : hdlBasic/Shift  shift_dir=Left  shift_bits=8  en=on  latency=1  precision=Full  arith_type="Signed  (2's comp)"  n_bits=16  bin_pt=14  quantization=Truncate  overflow=Wrap  XmcBlockStatus=1  maskContainerNames=group2  block_type=shift  block_config=sysgen:Shift_config
  Shift2 : hdlBasic/Shift  shift_dir=Left  shift_bits=1  en=on  latency=1  precision=Full  arith_type="Signed  (2's comp)"  n_bits=16  bin_pt=14  quantization=Truncate  overflow=Wrap  XmcBlockStatus=1  maskContainerNames=group2  block_type=shift  block_config=sysgen:Shift_config
  Shift3 : hdlBasic/Shift  shift_dir=Left  shift_bits=2  en=on  latency=1  precision=Full  arith_type="Signed  (2's comp)"  n_bits=16  bin_pt=14  quantization=Truncate  overflow=Wrap  XmcBlockStatus=1  maskContainerNames=group2  block_type=shift  block_config=sysgen:Shift_config
  Shift4 : hdlBasic/Shift  shift_dir=Left  shift_bits=3  en=on  latency=1  precision=Full  arith_type="Signed  (2's comp)"  n_bits=16  bin_pt=14  quantization=Truncate  overflow=Wrap  XmcBlockStatus=1  maskContainerNames=group2  block_type=shift  block_config=sysgen:Shift_config
  Shift5 : hdlBasic/Shift  shift_dir=Left  shift_bits=4  en=on  latency=1  precision=Full  arith_type="Signed  (2's comp)"  n_bits=16  bin_pt=14  quantization=Truncate  overflow=Wrap  XmcBlockStatus=1  maskContainerNames=group2  block_type=shift  block_config=sysgen:Shift_config
  Shift6 : hdlBasic/Shift  shift_dir=Left  shift_bits=5  en=on  latency=1  precision=Full  arith_type="Signed  (2's comp)"  n_bits=16  bin_pt=14  quantization=Truncate  overflow=Wrap  XmcBlockStatus=1  maskContainerNames=group2  block_type=shift  block_config=sysgen:Shift_config
  Shift7 : hdlBasic/Shift  shift_dir=Left  shift_bits=6  en=on  latency=1  precision=Full  arith_type="Signed  (2's comp)"  n_bits=16  bin_pt=14  quantization=Truncate  overflow=Wrap  XmcBlockStatus=1  maskContainerNames=group2  block_type=shift  block_config=sysgen:Shift_config
  Shift8 : hdlBasic/Shift  shift_dir=Left  shift_bits=7  en=on  latency=1  precision=Full  arith_type="Signed  (2's comp)"  n_bits=16  bin_pt=14  quantization=Truncate  overflow=Wrap  XmcBlockStatus=1  maskContainerNames=group2  block_type=shift  block_config=sysgen:Shift_config
  Shift9 : hdlBasic/Shift  shift_dir=Left  shift_bits=0  en=on  latency=1  precision=Full  arith_type="Signed  (2's comp)"  n_bits=16  bin_pt=14  quantization=Truncate  overflow=Wrap  XmcBlockStatus=1  maskContainerNames=group2  block_type=shift  block_config=sysgen:Shift_config
  Slice1 : hdlBasic/Slice  nbits=B  boolean_output=off  mode=Upper Bit Location + Width  bit1=0  base1=MSB of Input  bit0=8  base0=LSB of Input  XmcBlockStatus=1  maskContainerNames=group1  block_type=slice  block_config=sysgen:Slice_config
  v_out : Outport
  n_shift_out : Outport  Port=2
  mem_addr : Outport  Port=3
  wires:
  Shift7/1 -> Mux/8
  Shift4/1 -> Mux/5
  Shift6/1 -> Mux/7
  Shift2/1 -> Mux/3
  Shift8/1 -> Mux/9
  Shift3/1 -> Mux/4
  Shift5/1 -> Mux/6
  Slice1/1 -> mem_addr/1
  Shift1/1 -> Mux/10
  v_in/1 -> Shift1/1, Shift8/1, Shift7/1, Shift6/1, Shift5/1, Shift4/1, Shift3/1, Shift2/1, Shift9/1, Slice1/1
  Mux/1 -> v_out/1
  AddSub1/1 -> n_shift_out/1
  n_shift_in/1 -> Delay2/1
  mem_data_in/1 -> AddSub1/2, Mux/1
  Delay2/1 -> AddSub1/1
  Shift9/1 -> Mux/2
  en/1 -> Shift7/2, Shift6/2, Shift5/2, Shift4/2, Shift3/2, Shift2/2, Mux/11, AddSub1/3, Delay2/2, Shift9/2, Shift8/2, Shift1/2

== system env_extQ32/env_extr/SWT/shannonE/log2/normalize_input/stage3 ==
  v_in : Inport
  n_shift_in : Inport  Port=2
  mem_data_in : Inport  Port=3
  en : Inport  Port=4
  AddSub1 : hdlBasic/AddSub  mode=Addition  use_carryin=off  use_carryout=off  en=on  latency=1  precision=Full  arith_type=Unsigned  n_bits=16  bin_pt=14  quantization=Truncate  overflow=Wrap  use_behavioral_HDL=off  hw_selection=Fabric  pipelined=off  XmcBlockStatus=1  maskContainerNames=tabcontainer1  block_type=addsub  block_config=sysgen:Addsub_config
  Delay2 : hdlBasic/Delay  rst=off  en=on  latency=1  reg_retiming=off  XmcBlockStatus=1  maskContainerNames=group1  block_type=delay  block_config=sysgen:Delay_config
  Mux : hdlBasic/Mux  inputs=9  en=on  latency=1  precision=Full  arith_type=Unsigned  n_bits=16  bin_pt=14  quantization=Truncate  overflow=Wrap  XmcBlockStatus=1  maskContainerNames=tabcontainer1  block_type=mux  block_config=sysgen:Mux_config
  Shift1 : hdlBasic/Shift  shift_dir=Left  shift_bits=8  en=on  latency=1  precision=Full  arith_type="Signed  (2's comp)"  n_bits=16  bin_pt=14  quantization=Truncate  overflow=Wrap  XmcBlockStatus=1  maskContainerNames=group2  block_type=shift  block_config=sysgen:Shift_config
  Shift2 : hdlBasic/Shift  shift_dir=Left  shift_bits=1  en=on  latency=1  precision=Full  arith_type="Signed  (2's comp)"  n_bits=16  bin_pt=14  quantization=Truncate  overflow=Wrap  XmcBlockStatus=1  maskContainerNames=group2  block_type=shift  block_config=sysgen:Shift_config
  Shift3 : hdlBasic/Shift  shift_dir=Left  shift_bits=2  en=on  latency=1  precision=Full  arith_type="Signed  (2's comp)"  n_bits=16  bin_pt=14  quantization=Truncate  overflow=Wrap  XmcBlockStatus=1  maskContainerNames=group2  block_type=shift  block_config=sysgen:Shift_config
  Shift4 : hdlBasic/Shift  shift_dir=Left  shift_bits=3  en=on  latency=1  precision=Full  arith_type="Signed  (2's comp)"  n_bits=16  bin_pt=14  quantization=Truncate  overflow=Wrap  XmcBlockStatus=1  maskContainerNames=group2  block_type=shift  block_config=sysgen:Shift_config
  Shift5 : hdlBasic/Shift  shift_dir=Left  shift_bits=4  en=on  latency=1  precision=Full  arith_type="Signed  (2's comp)"  n_bits=16  bin_pt=14  quantization=Truncate  overflow=Wrap  XmcBlockStatus=1  maskContainerNames=group2  block_type=shift  block_config=sysgen:Shift_config
  Shift6 : hdlBasic/Shift  shift_dir=Left  shift_bits=5  en=on  latency=1  precision=Full  arith_type="Signed  (2's comp)"  n_bits=16  bin_pt=14  quantization=Truncate  overflow=Wrap  XmcBlockStatus=1  maskContainerNames=group2  block_type=shift  block_config=sysgen:Shift_config
  Shift7 : hdlBasic/Shift  shift_dir=Left  shift_bits=6  en=on  latency=1  precision=Full  arith_type="Signed  (2's comp)"  n_bits=16  bin_pt=14  quantization=Truncate  overflow=Wrap  XmcBlockStatus=1  maskContainerNames=group2  block_type=shift  block_config=sysgen:Shift_config
  Shift8 : hdlBasic/Shift  shift_dir=Left  shift_bits=7  en=on  latency=1  precision=Full  arith_type="Signed  (2's comp)"  n_bits=16  bin_pt=14  quantization=Truncate  overflow=Wrap  XmcBlockStatus=1  maskContainerNames=group2  block_type=shift  block_config=sysgen:Shift_config
  Shift9 : hdlBasic/Shift  shift_dir=Left  shift_bits=0  en=on  latency=1  precision=Full  arith_type="Signed  (2's comp)"  n_bits=16  bin_pt=14  quantization=Truncate  overflow=Wrap  XmcBlockStatus=1  maskContainerNames=group2  block_type=shift  block_config=sysgen:Shift_config
  Slice1 : hdlBasic/Slice  nbits=B  boolean_output=off  mode=Upper Bit Location + Width  bit1=0  base1=MSB of Input  bit0=8  base0=LSB of Input  XmcBlockStatus=1  maskContainerNames=group1  block_type=slice  block_config=sysgen:Slice_config
  v_out : Outport
  n_shift_out : Outport  Port=2
  mem_addr : Outport  Port=3
  wires:
  Shift7/1 -> Mux/8
  Shift4/1 -> Mux/5
  Shift6/1 -> Mux/7
  Shift2/1 -> Mux/3
  Shift8/1 -> Mux/9
  Shift3/1 -> Mux/4
  Shift5/1 -> Mux/6
  Slice1/1 -> mem_addr/1
  Shift1/1 -> Mux/10
  v_in/1 -> Shift1/1, Shift8/1, Shift7/1, Shift6/1, Shift5/1, Shift4/1, Shift3/1, Shift2/1, Shift9/1, Slice1/1
  Mux/1 -> v_out/1
  AddSub1/1 -> n_shift_out/1
  n_shift_in/1 -> Delay2/1
  mem_data_in/1 -> AddSub1/2, Mux/1
  Delay2/1 -> AddSub1/1
  Shift9/1 -> Mux/2
  en/1 -> Shift7/2, Shift6/2, Shift5/2, Shift4/2, Shift3/2, Shift2/2, Mux/11, AddSub1/3, Delay2/2, Shift9/2, Shift8/2, Shift1/2
